simulink model "MSAP"  (R2015a)
settings: Solver=ode3  StartTime=0.0  StopTime=2  FixedStep=Ts  RelTol=1e-3
values from neighbouring files (symbols this model uses):
  Ka = fluxeff    (= 0.15)    [VOC_param.m]    (also in VOC_param_paper.m; power_control_param.m)
  Ls = 2.7e-3    (= 0.0027)    [power_control_param.m]
  p = 4    [VOC_param.m]    (also in VOC_param_paper.m; power_control_param.m)
  rpm2radps = pi/30    (= 0.10471975512)    [VOC_param.m]    (also in VOC_param_paper.m; power_control_param.m)
  Rs = 1.137    [power_control_param.m]
settings Model: Creator=rblan  LastModifiedBy=rblan

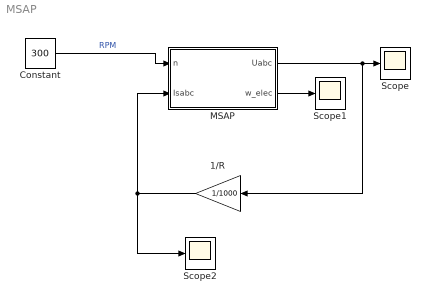
== system MSAP ==
  1/R : Gain  Gain=1/1000
  Constant : Constant  Value=300
  MSAP : Subsystem
  Scope : Scope
  Scope1 : Scope
  Scope2 : Scope
      settings: SaveName=ScopeData2
  wires:
  Constant/1 -> MSAP/1(n)  "RPM"
  MSAP/1(Uabc) -> 1/R/1, Scope/1
  MSAP/2(w_elec) -> Scope1/1
  1/R/1 -> Scope2/1, MSAP/2(Isabc)

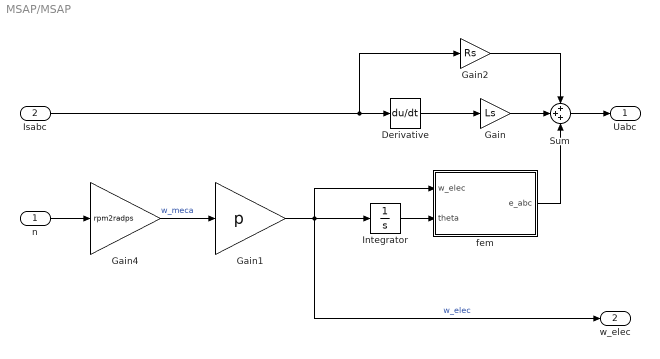
== system MSAP/MSAP ==
  n : Inport
  Isabc : Inport  Port=2
  Derivative : Derivative
  Gain : Gain  Gain=Ls
  Gain1 : Gain  Gain=p
  Gain2 : Gain  Gain=Rs
  Gain4 : Gain  Gain=rpm2radps
  Integrator : Integrator
  Sum : Sum  Inputs=+++
  fem : Subsystem
  Uabc : Outport
  w_elec : Outport  Port=2
  wires:
  Sum/1 -> Uabc/1
  Gain4/1 -> Gain1/1  "w_meca"
  n/1 -> Gain4/1
  Gain1/1 -> fem/1(w_elec), w_elec/1, Integrator/1  "w_elec"
  Integrator/1 -> fem/2(theta)
  Isabc/1 -> Gain2/1, Derivative/1
  Derivative/1 -> Gain/1
  Gain2/1 -> Sum/1
  Gain/1 -> Sum/2
  fem/1(e_abc) -> Sum/3

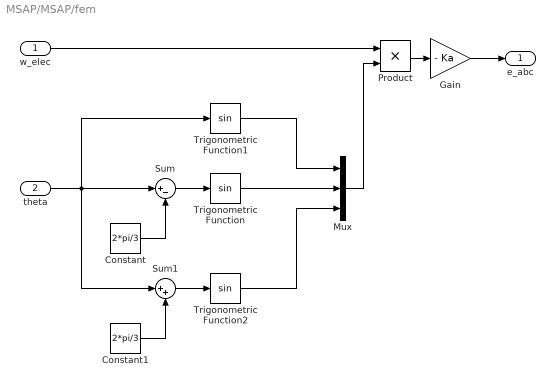
== system MSAP/MSAP/fem ==
  w_elec : Inport
  theta : Inport  Port=2
  Constant : Constant  Value=2*pi/3
  Constant1 : Constant  Value=2*pi/3
  Gain : Gain  Gain=- Ka
  Mux : Mux  Inputs=3
  Product : Product
  Sum : Sum  Inputs=|+-
  Sum1 : Sum  Inputs=|++
  Trigonometric Function : Trigonometry
  Trigonometric Function1 : Trigonometry
  Trigonometric Function2 : Trigonometry
  e_abc : Outport
  wires:
  Gain/1 -> e_abc/1
  Product/1 -> Gain/1
  w_elec/1 -> Product/1
  Sum/1 -> Trigonometric Function/1
  Constant/1 -> Sum/2
  Sum1/1 -> Trigonometric Function2/1
  Constant1/1 -> Sum1/2
  theta/1 -> Sum1/1, Trigonometric Function1/1, Sum/1
  Trigonometric Function1/1 -> Mux/1
  Trigonometric Function/1 -> Mux/2
  Trigonometric Function2/1 -> Mux/3
  Mux/1 -> Product/2
